simulink model "heatcool6"  (Simulink 5.0)
settings: Solver=ode45  StartTime=0.0  StopTime=TT(end)*Ts  RelTol=1e-3
values from neighbouring files (symbols this model uses):
  C = hybcon(S,Q,N,limits,refs)    [binary_inputs_sim.m]    (also in bm99benchmark.m; bm99norm2.m; bm99sim.m; exp2mld_mimo.m = lincon(model,'track',cost,interval,limits))
  P = pwa(S)    [bball.m]    (also in bm99sim.m; heatcool.m; logicstatesim.m; supply_chain.m)
libraries: hyblib x2
settings Model: LastModifiedBy=Alberto Bemporad  RTWOptions="-aEnforceIntegerDowncast=1 -aFoldNonRolledExpr=1 -aInlineInvariantSignals=1 -aInlineParameters=0 -aLocalBlockOutputs=1 -aRollThreshold=5 -aGenerateReport=0 -aGenCodeOnly=0 -aRTWVerbose=1 -aIncludeHyperlinkInReport=0 -aLaunchReport=0 -aForceParamTrailComments=0 -aGenerateComments=1 -aIgnoreCustomStorageClasses=1 -aIncHierarchyInIds=0 -aMaxRTWIdLen=31 -aShowEliminatedStatements=0 -aPrefixModelToSubsysFcnNames=1 -aIncDataTypeInIds=0 -aInsertBlockDesc=0 -aSimulinkBlockComments=1 -aInlinedPrmAccess=\"Literals\"  -aSuppressErrorStatus=0 -aModelReferenceCompliant=1 -aSupportNonInlinedSFcns=1 -aSupportContinuousTime=1 -aSupportComplex=1 -aSupportNonFinite=1 -aSupportAbsoluteTime=1 -aTargetPreCompLibLocation=\"\" -aTargetLibSuffix=\"\" -aTargetFcnLib=\"ansi_tfl_tmw.mat\" -aMultiInstanceERTCode=0 -aLogVarNameModifier=\"rt_\" -aIsPILTarget=0 -aCombineOutputUpdateFcns=0 -aGenerateASAP2=0 -aGenerateSampleERTMain=0 -aGenerateFullHeader=1 -aUtilityFuncGeneration=\"Auto\" -aIncludeFileDelimiter=\"Auto\" -aIncludeMdlTerminateFcn=1 -aPurelyIntegerCode=0 -aERTCustomFileBanners=0 -aRTWCAPIStates=0 -aRTWCAPIParams=0 -aRTWCAPISignals=0 -aMatFileLogging=1 -aGenFloatMathFcnCalls=\"ANSI_C\" -aExtModeMexFile=\"ext_comm\" -aExtModeTransport=0 -aExtModeStaticAllocSize=1000000 -aExtModeTesting=0 -aExtModeStaticAlloc=0 -aExtMode=0"

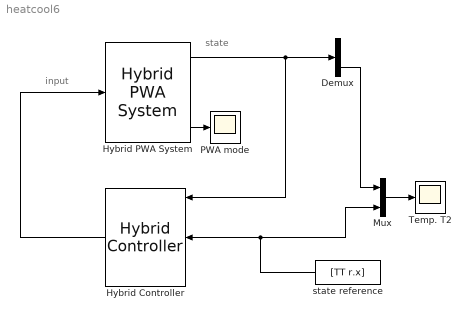
== system heatcool6 ==
  note: state
  note: input
  Demux : Demux  Outputs=2
  Hybrid Controller : hyblib/Hybrid Controller  Orientation=left  C=C  S=S
  Hybrid PWA System : hyblib/Hybrid PWA System  P=P  x0init=x0
  Mux : Mux  Inputs=2
  PWA mode : Scope
      settings: TimeRange=10  YMin=0  YMax=6  SaveName=ScopeData3
  Temp. T2 : Scope
      settings: TimeRange=50  YMin=0  YMax=50
  state reference : FromWorkspace  Orientation=left  VariableName=[TT r.x]
  wires:
  Hybrid PWA System/1 -> Hybrid Controller/1, Demux/1
  Hybrid PWA System/3 -> PWA mode/1
  state reference/1 -> Hybrid Controller/3, Mux/2
  Hybrid Controller/1 -> Hybrid PWA System/1
  Demux/2 -> Mux/1
  Mux/1 -> Temp. T2/1
